simulink model "NM100A_MotVelCtrl"  (R2013b)
settings: Solver=FixedStepDiscrete  SolverMode=SingleTasking  StartTime=0.0  StopTime=1  FixedStep=0.002  RelTol=1e-3
values from neighbouring files (symbols this model uses):
  ARCHGLBPRM_2MILLISEC_SEC_F32 = DataDict.Constant    [NM100A_MotVelCtrl_DataDict.m]
  DERIVTVLPFILTICONLOWRLIM_SEC_F32 = DataDict.Constant    [NM100A_MotVelCtrl_DataDict.m]
  FALSE_CNT_LGC = DataDict.Constant    [NM100A_MotVelCtrl_DataDict.m]
  MOTVELTHDRAMPDWNCMPL_MOTRADPERSEC_F32 = DataDict.Constant    [NM100A_MotVelCtrl_DataDict.m]
  ONEMILLISEC_SEC_F32 = DataDict.Constant    [NM100A_MotVelCtrl_DataDict.m]
  TITHDRAMPDWNCMPL_CNT_U16 = DataDict.Constant    [NM100A_MotVelCtrl_DataDict.m]
  TRUE_CNT_LGC = DataDict.Constant    [NM100A_MotVelCtrl_DataDict.m]
  ZEROMOTVELTAR_MOTRADPERSEC_F32 = DataDict.Constant    [NM100A_MotVelCtrl_DataDict.m]
  ZEROTQCMD_MOTNWTMTR_F32 = DataDict.Constant    [NM100A_MotVelCtrl_DataDict.m]
libraries: NxtrLim x13, simulink x1, NxtrAbslt x1, NxtrMax x1
(part 2 of 4)

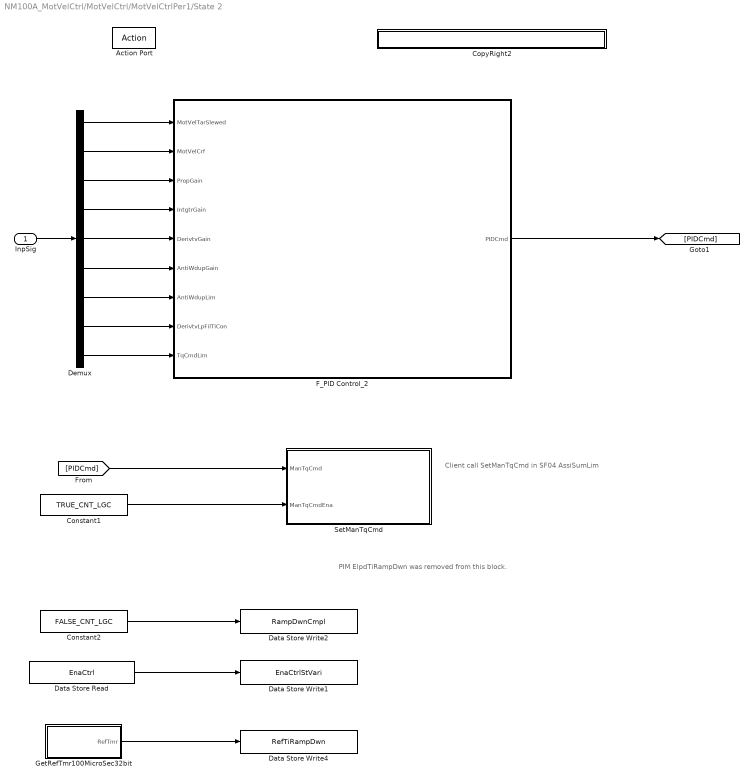
== system NM100A_MotVelCtrl/MotVelCtrl/MotVelCtrlPer1/State 2 ==
  note: PIM ElpdTiRampDwn was removed from this block.
  note: Client call SetManTqCmd in SF04 AssiSumLim
  "InpSig " : Inport
  Action Port : ActionPort  ActionType=elseif
  Constant1 : Constant  RequirementInfo="{'linktype_rmi_doors' '00010020 (/E-STEER Core/SubSystem Specifications/Manufacturing Service/NM100A_Motor Velocity Control Function Requirement)' '#NM100A_49' 'true' 'REQ:  NM100A_49' '' } %GIDa_befda8d9_aa94_48ad_b962_3d809fb1409c"  Value=TRUE_CNT_LGC
  Constant2 : Constant  RequirementInfo="{'linktype_rmi_doors' '00010020 (/E-STEER Core/SubSystem Specifications/Manufacturing Service/NM100A_Motor Velocity Control Function Requirement)' '#NM100A_49' 'true' 'REQ:  NM100A_49' '' } %GIDa_4dd34f10_b749_44c9_b696_3da1388302c2"  Value=FALSE_CNT_LGC
  CopyRight2 : Subsystem  Description=|  mask(Copyright Information){none=on}
      | Copyright info block.                                               
      |                                                                     
      | Place copyright information at the top of every subsystem in design.
      mask prompts: none "No parameters"
      mask help: Place copyright information at the top of every subsystem in design.
      mask Display:
      | NxtrConf = 'Nexteer Confidential';
      | 
      | sys = bdroot; %handle for the current model ("system")
      | first = get_param(sys,'Created');
      | if(isempty(first))
      |     first = datestr(now,'yyyy');
      | else
      |     first = first(end-3:end);  %year is last four digits
      | end
      | 
      | last = get_param(sys,'LastModifiedDate');
      | if isempty(last)
      |     last = datestr(now,'yyyy');
      | else
      |     last = last(end-3:end);
      | end
      | 
      | if strcmp(first,last)
      |     fprintf('%s -- Copyright %s Nexteer',NxtrConf,first)
      | else
      |     fprintf('%s -- %s%s- %s Nexteer',NxtrConf,char(169),first,last)
      | end
  Data Store Read : DataStoreRead  RequirementInfo={} %GIDa_be0bc7da_d338_4404_a31b_81b9c0ca05c9  DataStoreName=EnaCtrl
  Data Store Write1 : DataStoreWrite  RequirementInfo={} %GIDa_9c211729_4960_4e3d_a14f_2673763a524a  DataStoreName=EnaCtrlStVari
  Data Store Write2 : DataStoreWrite  RequirementInfo="{'linktype_rmi_doors' '00010020 (/E-STEER Core/SubSystem Specifications/Manufacturing Service/NM100A_Motor Velocity Control Function Requirement)' '#NM100A_49' 'true' 'REQ:  NM100A_49' '' ; 'linktype_rmi_doors' '00010020 (/E-STEER Core/SubSystem Specifications/Manufacturing Service/NM100A_Motor Velocity Control Function Requirement)' '#NM100A_49' 'true' 'REQ:  NM100A_49' '' } %GIDa_77af4ed3_6787_4830_bfc0_e32d42128aa7"  DataStoreName=RampDwnCmpl
  Data Store Write4 : DataStoreWrite  RequirementInfo="{'linktype_rmi_doors' '00010020 (/E-STEER Core/SubSystem Specifications/Manufacturing Service/NM100A_Motor Velocity Control Function Requirement)' '#NM100A_49' 'true' 'REQ:  NM100A_49' '' } %GIDa_d0b5b3f8_5505_4299_b70c_b09a5e077bdf"  DataStoreName=RefTiRampDwn
  Demux : Demux  Outputs=9
  F_PID Control_2 : Subsystem
  GetRefTmr100MicroSec32bit : Subsystem  RequirementInfo="{'linktype_rmi_doors' '00010020 (/E-STEER Core/SubSystem Specifications/Manufacturing Service/NM100A_Motor Velocity Control Function Requirement)' '#NM100A_49' 'true' 'REQ:  NM100A_49' '' } %GIDa_d3dda55e_dd8c_4cb5_ad41_cdb42cb83704"
  SetManTqCmd : Subsystem  RequirementInfo={} %GIDa_d5276b83_f182_4895_b3b8_b6924f7a4ac8
  wires:
  Data Store Read/1 -> Data Store Write1/1
  Constant1/1 -> SetManTqCmd/2(ManTqCmdEna)
  [PIDCmd] -> SetManTqCmd/1(ManTqCmd)
  Constant2/1 -> Data Store Write2/1
  GetRefTmr100MicroSec32bit/1(RefTmr) -> Data Store Write4/1
  F_PID Control_2/1("PIDCmd ") -> [PIDCmd]
  "InpSig "/1 -> Demux/1
  Demux/9 -> F_PID Control_2/9(TqCmdLim)
  Demux/8 -> F_PID Control_2/8(DerivtvLpFilTiCon)
  Demux/1 -> F_PID Control_2/1(MotVelTarSlewed)
  Demux/2 -> F_PID Control_2/2(MotVelCrf)
  Demux/3 -> F_PID Control_2/3(PropGain)
  Demux/4 -> F_PID Control_2/4(IntgtrGain)
  Demux/5 -> F_PID Control_2/5(DerivtvGain)
  Demux/6 -> F_PID Control_2/6(AntiWdupGain)
  Demux/7 -> F_PID Control_2/7(AntiWdupLim)

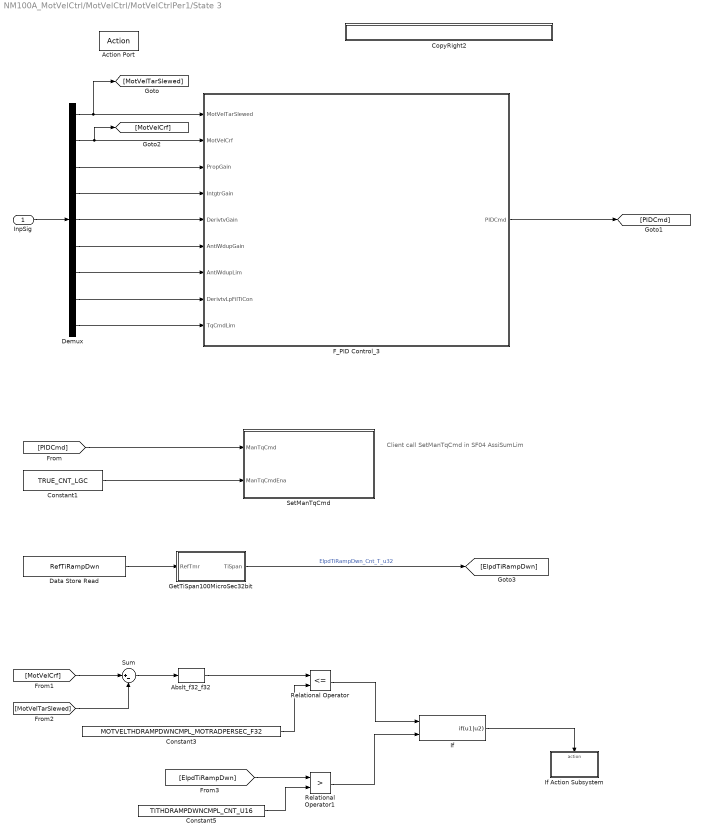
== system NM100A_MotVelCtrl/MotVelCtrl/MotVelCtrlPer1/State 3 ==
  note: Client call SetManTqCmd in SF04 AssiSumLim
  "InpSig " : Inport
  Action Port : ActionPort  ActionType=elseif
  Abslt_f32_f32 : NxtrAbslt/Abslt_f32_f32  RequirementInfo="{'linktype_rmi_doors' '00010020 (/E-STEER Core/SubSystem Specifications/Manufacturing Service/NM100A_Motor Velocity Control Function Requirement)' '#NM100A_102' 'true' 'REQ:  NM100A_102' '' } %GIDa_71536a81_3999_4725_b831_59cc761146c6"  SFunctionSpec=single y1 = Abslt_f32_f32(single u1)
      settings: AttributesFormatString=%<Name>
  Constant1 : Constant  RequirementInfo="{'linktype_rmi_doors' '00010020 (/E-STEER Core/SubSystem Specifications/Manufacturing Service/NM100A_Motor Velocity Control Function Requirement)' '#NM100A_51' 'true' 'REQ:  NM100A_51' '' } %GIDa_145580c1_2ef8_4b58_be2f_cd9335f096b6"  Value=TRUE_CNT_LGC
  Constant3 : Constant  RequirementInfo="{'linktype_rmi_doors' '00010020 (/E-STEER Core/SubSystem Specifications/Manufacturing Service/NM100A_Motor Velocity Control Function Requirement)' '#NM100A_102' 'true' 'REQ:  NM100A_102' '' } %GIDa_e1d28c76_b859_4531_ad36_30c270ff2bb5"  Value=MOTVELTHDRAMPDWNCMPL_MOTRADPERSEC_F32
  Constant5 : Constant  RequirementInfo="{'linktype_rmi_doors' '00010020 (/E-STEER Core/SubSystem Specifications/Manufacturing Service/NM100A_Motor Velocity Control Function Requirement)' '#NM100A_102' 'true' 'REQ:  NM100A_102' '' } %GIDa_b4be8dec_013e_43ed_818c_6b151e6f5195"  Value=TITHDRAMPDWNCMPL_CNT_U16
  CopyRight2 : Subsystem  Description=|  mask(Copyright Information){none=on}
      | Copyright info block.                                               
      |                                                                     
      | Place copyright information at the top of every subsystem in design.
      mask prompts: none "No parameters"
      mask help: Place copyright information at the top of every subsystem in design.
      mask Display:
      | NxtrConf = 'Nexteer Confidential';
      | 
      | sys = bdroot; %handle for the current model ("system")
      | first = get_param(sys,'Created');
      | if(isempty(first))
      |     first = datestr(now,'yyyy');
      | else
      |     first = first(end-3:end);  %year is last four digits
      | end
      | 
      | last = get_param(sys,'LastModifiedDate');
      | if isempty(last)
      |     last = datestr(now,'yyyy');
      | else
      |     last = last(end-3:end);
      | end
      | 
      | if strcmp(first,last)
      |     fprintf('%s -- Copyright %s Nexteer',NxtrConf,first)
      | else
      |     fprintf('%s -- %s%s- %s Nexteer',NxtrConf,char(169),first,last)
      | end
  Data Store Read : DataStoreRead  RequirementInfo="{'linktype_rmi_doors' '00010020 (/E-STEER Core/SubSystem Specifications/Manufacturing Service/NM100A_Motor Velocity Control Function Requirement)' '#NM100A_51' 'true' 'REQ:  NM100A_51' '' } %GIDa_01a06484_7057_4d5d_9dfb_f9d8c90e0876"  DataStoreName=RefTiRampDwn
  Demux : Demux  Outputs=9
  F_PID Control_3 : Subsystem
  GetTiSpan100MicroSec32bit : Subsystem  RequirementInfo="{'linktype_rmi_doors' '00010020 (/E-STEER Core/SubSystem Specifications/Manufacturing Service/NM100A_Motor Velocity Control Function Requirement)' '#NM100A_51' 'true' 'REQ:  NM100A_51' '' } %GIDa_c327af38_75a4_49ae_9dcc_6e10e32790a8"
  If : If  RequirementInfo="{'linktype_rmi_doors' '00010020 (/E-STEER Core/SubSystem Specifications/Manufacturing Service/NM100A_Motor Velocity Control Function Requirement)' '#NM100A_102' 'true' 'REQ:  NM100A_102' '' } %GIDa_380769d0_dc6b_456e_a037_bb1d2f196c72"  NumInputs=2  IfExpression=u1|u2  ShowElse=off
  If Action Subsystem : Subsystem  RequirementInfo="{'linktype_rmi_doors' '00010020 (/E-STEER Core/SubSystem Specifications/Manufacturing Service/NM100A_Motor Velocity Control Function Requirement)' '#NM100A_102' 'true' 'REQ:  NM100A_102' '' } %GIDa_fba956b4_c918_457d_ab20_4a25f3a425a7"  TreatAsAtomicUnit=on
  Relational Operator : RelationalOperator  RequirementInfo="{'linktype_rmi_doors' '00010020 (/E-STEER Core/SubSystem Specifications/Manufacturing Service/NM100A_Motor Velocity Control Function Requirement)' '#NM100A_102' 'true' 'REQ:  NM100A_102' '' } %GIDa_1c0824c1_3317_422e_9fa2_aea2872f56e4"  Operator=<=  OutDataTypeStr=boolean
  Relational Operator1 : RelationalOperator  RequirementInfo="{'linktype_rmi_doors' '00010020 (/E-STEER Core/SubSystem Specifications/Manufacturing Service/NM100A_Motor Velocity Control Function Requirement)' '#NM100A_102' 'true' 'REQ:  NM100A_102' '' } %GIDa_87284f63_b176_4ff1_b10d_fd7dc0737078"  Operator=>  OutDataTypeStr=boolean
  SetManTqCmd : Subsystem  RequirementInfo={} %GIDa_e23fb978_d226_45a3_bc03_4908240c5a9f
  Sum : Sum  RequirementInfo="{'linktype_rmi_doors' '00010020 (/E-STEER Core/SubSystem Specifications/Manufacturing Service/NM100A_Motor Velocity Control Function Requirement)' '#NM100A_102' 'true' 'REQ:  NM100A_102' '' } %GIDa_50c60e5b_59b9_4476_b7b5_e8ccd2770148"  Inputs=|+-
  wires:
  GetTiSpan100MicroSec32bit/1(TiSpan) -> [ElpdTiRampDwn]  "ElpdTiRampDwn_Cnt_T_u32"
  Data Store Read/1 -> GetTiSpan100MicroSec32bit/1(RefTmr)
  [MotVelCrf] -> Sum/1
  [MotVelTarSlewed] -> Sum/2
  Sum/1 -> Abslt_f32_f32/1
  Abslt_f32_f32/1 -> Relational Operator/1
  Constant3/1 -> Relational Operator/2
  [ElpdTiRampDwn] -> Relational Operator1/1
  Constant5/1 -> Relational Operator1/2
  Relational Operator/1 -> If/1
  Relational Operator1/1 -> If/2
  If/1 -> If Action Subsystem/Action
  [PIDCmd] -> SetManTqCmd/1(ManTqCmd)
  Constant1/1 -> SetManTqCmd/2(ManTqCmdEna)
  F_PID Control_3/1("PIDCmd ") -> [PIDCmd]
  "InpSig "/1 -> Demux/1
  Demux/9 -> F_PID Control_3/9(TqCmdLim)
  Demux/8 -> F_PID Control_3/8(DerivtvLpFilTiCon)
  Demux/1 -> [MotVelTarSlewed], F_PID Control_3/1(MotVelTarSlewed)
  Demux/2 -> [MotVelCrf], F_PID Control_3/2(MotVelCrf)
  Demux/3 -> F_PID Control_3/3(PropGain)
  Demux/4 -> F_PID Control_3/4(IntgtrGain)
  Demux/5 -> F_PID Control_3/5(DerivtvGain)
  Demux/6 -> F_PID Control_3/6(AntiWdupGain)
  Demux/7 -> F_PID Control_3/7(AntiWdupLim)

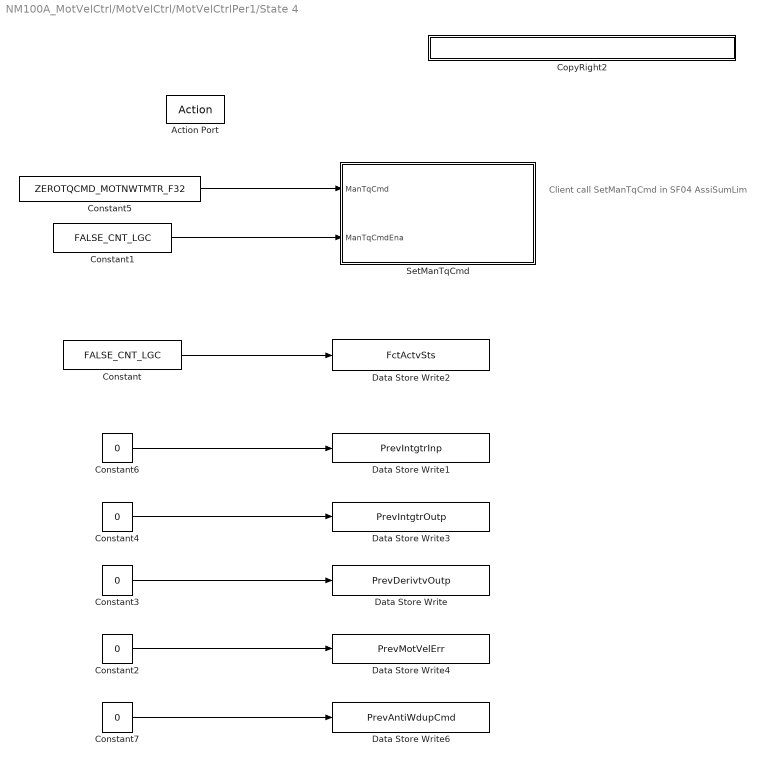
== system NM100A_MotVelCtrl/MotVelCtrl/MotVelCtrlPer1/State 4 ==
  note: Client call SetManTqCmd in SF04 AssiSumLim
  Action Port : ActionPort  ActionType=elseif
  Constant : Constant  RequirementInfo="{'linktype_rmi_doors' '00010020 (/E-STEER Core/SubSystem Specifications/Manufacturing Service/NM100A_Motor Velocity Control Function Requirement)' '#NM100A_103' 'true' 'REQ:  NM100A_103' '' } %GIDa_e0af5cdd_08fc_4257_96fd_548f729c1ff8"  Value=FALSE_CNT_LGC
  Constant1 : Constant  RequirementInfo="{'linktype_rmi_doors' '00010020 (/E-STEER Core/SubSystem Specifications/Manufacturing Service/NM100A_Motor Velocity Control Function Requirement)' '#NM100A_103' 'true' 'REQ:  NM100A_103' '' } %GIDa_4a98490f_aa1d_4f3d_87f2_701335d2a890"  Value=FALSE_CNT_LGC
  Constant2 : Constant  RequirementInfo="{'linktype_rmi_doors' '00010020 (/E-STEER Core/SubSystem Specifications/Manufacturing Service/NM100A_Motor Velocity Control Function Requirement)' '#NM100A_132' 'true' 'REQ:  NM100A_132' '' } %GIDa_c08df92f_5a02_4e06_8009_e26f95953966"  Value=0  OutDataTypeStr=single
  Constant3 : Constant  RequirementInfo="{'linktype_rmi_doors' '00010020 (/E-STEER Core/SubSystem Specifications/Manufacturing Service/NM100A_Motor Velocity Control Function Requirement)' '#NM100A_132' 'true' 'REQ:  NM100A_132' '' } %GIDa_74271fdc_8687_4593_ab71_e98823fce526"  Value=0  OutDataTypeStr=single
  Constant4 : Constant  RequirementInfo="{'linktype_rmi_doors' '00010020 (/E-STEER Core/SubSystem Specifications/Manufacturing Service/NM100A_Motor Velocity Control Function Requirement)' '#NM100A_132' 'true' 'REQ:  NM100A_132' '' } %GIDa_5f8c01d9_33ff_4742_87ff_920fa99edd06"  Value=0  OutDataTypeStr=single
  Constant5 : Constant  RequirementInfo="{'linktype_rmi_doors' '00010020 (/E-STEER Core/SubSystem Specifications/Manufacturing Service/NM100A_Motor Velocity Control Function Requirement)' '#NM100A_103' 'true' 'REQ:  NM100A_103' '' } %GIDa_14e8f590_79a8_40b3_b671_09126d55396b"  Value=ZEROTQCMD_MOTNWTMTR_F32
  Constant6 : Constant  RequirementInfo="{'linktype_rmi_doors' '00010020 (/E-STEER Core/SubSystem Specifications/Manufacturing Service/NM100A_Motor Velocity Control Function Requirement)' '#NM100A_132' 'true' 'REQ:  NM100A_132' '' } %GIDa_6c204c9d_6218_436f_9ecb_c10029247157"  Value=0  OutDataTypeStr=single
  Constant7 : Constant  RequirementInfo="{'linktype_rmi_doors' '00010020 (/E-STEER Core/SubSystem Specifications/Manufacturing Service/NM100A_Motor Velocity Control Function Requirement)' '#NM100A_132' 'true' 'REQ:  NM100A_132' '' } %GIDa_c396e5c7_5d94_4e94_a666_aede99a7520f"  Value=0  OutDataTypeStr=single
  CopyRight2 : Subsystem  Description=|  mask(Copyright Information){none=on}
      | Copyright info block.                                               
      |                                                                     
      | Place copyright information at the top of every subsystem in design.
      mask prompts: none "No parameters"
      mask help: Place copyright information at the top of every subsystem in design.
      mask Display:
      | NxtrConf = 'Nexteer Confidential';
      | 
      | sys = bdroot; %handle for the current model ("system")
      | first = get_param(sys,'Created');
      | if(isempty(first))
      |     first = datestr(now,'yyyy');
      | else
      |     first = first(end-3:end);  %year is last four digits
      | end
      | 
      | last = get_param(sys,'LastModifiedDate');
      | if isempty(last)
      |     last = datestr(now,'yyyy');
      | else
      |     last = last(end-3:end);
      | end
      | 
      | if strcmp(first,last)
      |     fprintf('%s -- Copyright %s Nexteer',NxtrConf,first)
      | else
      |     fprintf('%s -- %s%s- %s Nexteer',NxtrConf,char(169),first,last)
      | end
  Data Store Write : DataStoreWrite  RequirementInfo="{'linktype_rmi_doors' '00010020 (/E-STEER Core/SubSystem Specifications/Manufacturing Service/NM100A_Motor Velocity Control Function Requirement)' '#NM100A_132' 'true' 'REQ:  NM100A_132' '' } %GIDa_d60505be_a89c_40ef_ad23_4df5d7d8441f"  DataStoreName=PrevDerivtvOutp
  Data Store Write1 : DataStoreWrite  RequirementInfo="{'linktype_rmi_doors' '00010020 (/E-STEER Core/SubSystem Specifications/Manufacturing Service/NM100A_Motor Velocity Control Function Requirement)' '#NM100A_132' 'true' 'REQ:  NM100A_132' '' } %GIDa_90c6de6d_b636_45fd_be9c_0bef990974b9"  DataStoreName=PrevIntgtrInp
  Data Store Write2 : DataStoreWrite  RequirementInfo="{'linktype_rmi_doors' '00010020 (/E-STEER Core/SubSystem Specifications/Manufacturing Service/NM100A_Motor Velocity Control Function Requirement)' '#NM100A_103' 'true' 'REQ:  NM100A_103' '' } %GIDa_ce885f20_d047_4a81_96f7_7d088f6c7471"  DataStoreName=FctActvSts
  Data Store Write3 : DataStoreWrite  RequirementInfo="{'linktype_rmi_doors' '00010020 (/E-STEER Core/SubSystem Specifications/Manufacturing Service/NM100A_Motor Velocity Control Function Requirement)' '#NM100A_132' 'true' 'REQ:  NM100A_132' '' } %GIDa_cc8f8250_d580_4b1e_ba1d_46df9b018bff"  DataStoreName=PrevIntgtrOutp
  Data Store Write4 : DataStoreWrite  RequirementInfo="{'linktype_rmi_doors' '00010020 (/E-STEER Core/SubSystem Specifications/Manufacturing Service/NM100A_Motor Velocity Control Function Requirement)' '#NM100A_132' 'true' 'REQ:  NM100A_132' '' } %GIDa_fa392152_1c2a_4bda_84e9_c453589a09fe"  DataStoreName=PrevMotVelErr
  Data Store Write6 : DataStoreWrite  RequirementInfo="{'linktype_rmi_doors' '00010020 (/E-STEER Core/SubSystem Specifications/Manufacturing Service/NM100A_Motor Velocity Control Function Requirement)' '#NM100A_132' 'true' 'REQ:  NM100A_132' '' } %GIDa_e967ece6_5ffc_46ce_86f4_378f565c98d6"  DataStoreName=PrevAntiWdupCmd
  SetManTqCmd : Subsystem  RequirementInfo={} %GIDa_c501183d_31f0_413c_9518_9aa274485215
  wires:
  Constant/1 -> Data Store Write2/1
  Constant5/1 -> SetManTqCmd/1(ManTqCmd)
  Constant1/1 -> SetManTqCmd/2(ManTqCmdEna)
  Constant2/1 -> Data Store Write4/1
  Constant3/1 -> Data Store Write/1
  Constant4/1 -> Data Store Write3/1
  Constant6/1 -> Data Store Write1/1
  Constant7/1 -> Data Store Write6/1

== system NM100A_MotVelCtrl/MotVelCtrl/MotVelCtrlPer1/State 5 Do Nothing ==
  note: Wait and do nothing in this state.
  Action Port : ActionPort  ActionType=else
  CopyRight2 : Subsystem  Description=|  mask(Copyright Information){none=on}
      | Copyright info block.                                               
      |                                                                     
      | Place copyright information at the top of every subsystem in design.
      mask prompts: none "No parameters"
      mask help: Place copyright information at the top of every subsystem in design.
      mask Display:
      | NxtrConf = 'Nexteer Confidential';
      | 
      | sys = bdroot; %handle for the current model ("system")
      | first = get_param(sys,'Created');
      | if(isempty(first))
      |     first = datestr(now,'yyyy');
      | else
      |     first = first(end-3:end);  %year is last four digits
      | end
      | 
      | last = get_param(sys,'LastModifiedDate');
      | if isempty(last)
      |     last = datestr(now,'yyyy');
      | else
      |     last = last(end-3:end);
      | end
      | 
      | if strcmp(first,last)
      |     fprintf('%s -- Copyright %s Nexteer',NxtrConf,first)
      | else
      |     fprintf('%s -- %s%s- %s Nexteer',NxtrConf,char(169),first,last)
      | end

== system NM100A_MotVelCtrl/MotVelCtrl/SetCtrlPrm/CopyRight2 ==

== system NM100A_MotVelCtrl/MotVelCtrl/StopCtrl/CopyRight2 ==

== system NM100A_MotVelCtrl/MotVelCtrl/StrtCtrl/CopyRight2 ==

== system NM100A_MotVelCtrl/MotVelCtrl/MotVelCtrlPer1/SlewMotVelTar/CopyRight2 ==

== system NM100A_MotVelCtrl/MotVelCtrl/MotVelCtrlPer1/State 1/CopyRight2 ==

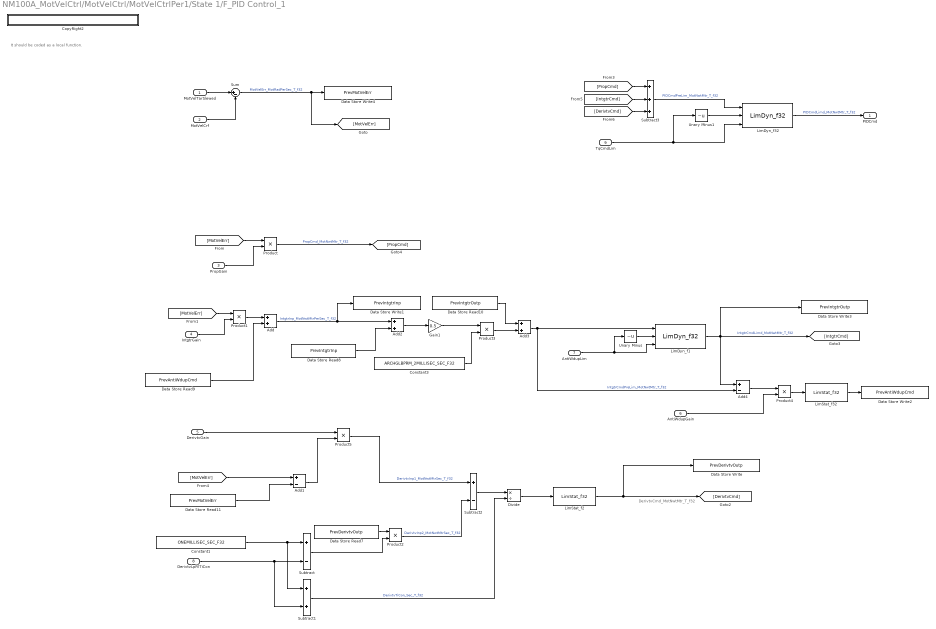
== system NM100A_MotVelCtrl/MotVelCtrl/MotVelCtrlPer1/State 1/F_PID Control_1 ==
  note: DerivtvCmd_MotNwtMtr_T_f32
  note: It should be coded as a local function.
  MotVelTarSlewed : Inport  RequirementInfo="{'linktype_rmi_doors' '00010020 (/E-STEER Core/SubSystem Specifications/Manufacturing Service/NM100A_Motor Velocity Control Function Requirement)' '#NM100A_30' 'true' 'REQ:  NM100A_30' '' } %GIDa_ba9429c3_b2a6_44fd_8328_ed63e261e922"
  MotVelCrf : Inport  RequirementInfo="{'linktype_rmi_doors' '00010020 (/E-STEER Core/SubSystem Specifications/Manufacturing Service/NM100A_Motor Velocity Control Function Requirement)' '#NM100A_30' 'true' 'REQ:  NM100A_30' '' } %GIDa_249e43ce_6396_4e5c_aa17_12a37b4ce850"  Port=2
  PropGain : Inport  RequirementInfo="{'linktype_rmi_doors' '00010020 (/E-STEER Core/SubSystem Specifications/Manufacturing Service/NM100A_Motor Velocity Control Function Requirement)' '#NM100A_112' 'true' 'REQ:  NM100A_112' '' } %GIDa_d2918d69_dd8c_483f_a043_c74a9c170ab9"  Port=3
  IntgtrGain : Inport  RequirementInfo="{'linktype_rmi_doors' '00010020 (/E-STEER Core/SubSystem Specifications/Manufacturing Service/NM100A_Motor Velocity Control Function Requirement)' '#NM100A_115' 'true' 'REQ:  NM100A_115' '' } %GIDa_bd070368_5372_458b_86f2_5ff06bf43677"  Port=4
  DerivtvGain : Inport  RequirementInfo="{'linktype_rmi_doors' '00010020 (/E-STEER Core/SubSystem Specifications/Manufacturing Service/NM100A_Motor Velocity Control Function Requirement)' '#NM100A_116' 'true' 'REQ:  NM100A_116' '' } %GIDa_947ca68e_fedf_47ef_844e_2f43d2f7ba60"  Port=5
  AntiWdupGain : Inport  RequirementInfo="{'linktype_rmi_doors' '00010020 (/E-STEER Core/SubSystem Specifications/Manufacturing Service/NM100A_Motor Velocity Control Function Requirement)' '#NM100A_118' 'true' 'REQ:  NM100A_118' '' } %GIDa_38b42111_2f7d_457c_8f7a_1eb8d27ba3f8"  Port=6
  AntiWdupLim : Inport  RequirementInfo="{'linktype_rmi_doors' '00010020 (/E-STEER Core/SubSystem Specifications/Manufacturing Service/NM100A_Motor Velocity Control Function Requirement)' '#NM100A_118' 'true' 'REQ:  NM100A_118' '' } %GIDa_29cfa6f2_eda7_4d1c_8a74_b9a9d786c745"  Port=7
  DerivtvLpFilTiCon : Inport  RequirementInfo="{'linktype_rmi_doors' '00010020 (/E-STEER Core/SubSystem Specifications/Manufacturing Service/NM100A_Motor Velocity Control Function Requirement)' '#NM100A_116' 'true' 'REQ:  NM100A_116' '' } %GIDa_5626f835_1586_4d6d_8f6e_8c5bf324693b"  Port=8
  TqCmdLim : Inport  RequirementInfo="{'linktype_rmi_doors' '00010020 (/E-STEER Core/SubSystem Specifications/Manufacturing Service/NM100A_Motor Velocity Control Function Requirement)' '#NM100A_123' 'true' 'REQ:  NM100A_123' '' } %GIDa_1e3e1849_4718_4d31_8f87_cac933a70f40"  Port=9
  Add : Sum  RequirementInfo="{'linktype_rmi_doors' '00010020 (/E-STEER Core/SubSystem Specifications/Manufacturing Service/NM100A_Motor Velocity Control Function Requirement)' '#NM100A_115' 'true' 'REQ:  NM100A_115' '' } %GIDa_25a704dd_c9d1_4845_b956_997790c43ace"
  Add1 : Sum  RequirementInfo="{'linktype_rmi_doors' '00010020 (/E-STEER Core/SubSystem Specifications/Manufacturing Service/NM100A_Motor Velocity Control Function Requirement)' '#NM100A_116' 'true' 'REQ:  NM100A_116' '' } %GIDa_012f7c69_ba98_4d6b_b5f0_33cfecf4ee6d"  Inputs=+-
  Add2 : Sum  RequirementInfo="{'linktype_rmi_doors' '00010020 (/E-STEER Core/SubSystem Specifications/Manufacturing Service/NM100A_Motor Velocity Control Function Requirement)' '#NM100A_115' 'true' 'REQ:  NM100A_115' '' } %GIDa_529e6f67_8be2_4dad_9470_b5eba2f52912"
  Add3 : Sum  RequirementInfo="{'linktype_rmi_doors' '00010020 (/E-STEER Core/SubSystem Specifications/Manufacturing Service/NM100A_Motor Velocity Control Function Requirement)' '#NM100A_115' 'true' 'REQ:  NM100A_115' '' } %GIDa_50298e16_fdb3_4c99_8cdc_cd68ad835e0b"
  Add4 : Sum  RequirementInfo={'linktype_rmi_doors' '00010020 (/E-STEER Core/SubSystem Specifications/Manufacturing Service/NM100A_Motor Velocity Control Function Requirement)' '#NM100A_118' 'true' 'REQ:NM100A_118' '' } %GIDa_b87562fd_2e83_4d37_9c91_b002b33c54af  Inputs=+-
  Constant1 : Constant  RequirementInfo="{'linktype_rmi_doors' '00010020 (/E-STEER Core/SubSystem Specifications/Manufacturing Service/NM100A_Motor Velocity Control Function Requirement)' '#NM100A_116' 'true' 'REQ:  NM100A_116' '' } %GIDa_70122f75_8c90_4f57_9e0f_909ebc7f7a2c"  Value=ONEMILLISEC_SEC_F32
  Constant3 : Constant  RequirementInfo="{'linktype_rmi_doors' '00010020 (/E-STEER Core/SubSystem Specifications/Manufacturing Service/NM100A_Motor Velocity Control Function Requirement)' '#NM100A_115' 'true' 'REQ:  NM100A_115' '' } %GIDa_9527d714_8fcf_4559_8899_418ffd3a7660"  Value=ARCHGLBPRM_2MILLISEC_SEC_F32
  CopyRight2 : Subsystem  Description=|  mask(Copyright Information){none=on}
      | Copyright info block.                                               
      |                                                                     
      | Place copyright information at the top of every subsystem in design.
      mask prompts: none "No parameters"
      mask help: Place copyright information at the top of every subsystem in design.
      mask Display:
      | NxtrConf = 'Nexteer Confidential';
      | 
      | sys = bdroot; %handle for the current model ("system")
      | first = get_param(sys,'Created');
      | if(isempty(first))
      |     first = datestr(now,'yyyy');
      | else
      |     first = first(end-3:end);  %year is last four digits
      | end
      | 
      | last = get_param(sys,'LastModifiedDate');
      | if isempty(last)
      |     last = datestr(now,'yyyy');
      | else
      |     last = last(end-3:end);
      | end
      | 
      | if strcmp(first,last)
      |     fprintf('%s -- Copyright %s Nexteer',NxtrConf,first)
      | else
      |     fprintf('%s -- %s%s- %s Nexteer',NxtrConf,char(169),first,last)
      | end
  Data Store Read10 : DataStoreRead  RequirementInfo="{'linktype_rmi_doors' '00010020 (/E-STEER Core/SubSystem Specifications/Manufacturing Service/NM100A_Motor Velocity Control Function Requirement)' '#NM100A_115' 'true' 'REQ:  NM100A_115' '' } %GIDa_687aece3_9f80_466d_9de9_e3cb1ea81850"  Priority=1  DataStoreName=PrevIntgtrOutp
  Data Store Read11 : DataStoreRead  RequirementInfo="{'linktype_rmi_doors' '00010020 (/E-STEER Core/SubSystem Specifications/Manufacturing Service/NM100A_Motor Velocity Control Function Requirement)' '#NM100A_116' 'true' 'REQ:  NM100A_116' '' } %GIDa_4290bcdf_0a17_42a8_9871_b33e1ea3d554"  Priority=1  DataStoreName=PrevMotVelErr
  Data Store Read7 : DataStoreRead  RequirementInfo="{'linktype_rmi_doors' '00010020 (/E-STEER Core/SubSystem Specifications/Manufacturing Service/NM100A_Motor Velocity Control Function Requirement)' '#NM100A_116' 'true' 'REQ:  NM100A_116' '' } %GIDa_d5aac981_534e_4fe9_8c13_af2e2de1b167"  Priority=1  DataStoreName=PrevDerivtvOutp
  Data Store Read8 : DataStoreRead  RequirementInfo="{'linktype_rmi_doors' '00010020 (/E-STEER Core/SubSystem Specifications/Manufacturing Service/NM100A_Motor Velocity Control Function Requirement)' '#NM100A_115' 'true' 'REQ:  NM100A_115' '' } %GIDa_a386e5fa_5ba8_459d_b678_d402aa374cd6"  Priority=1  DataStoreName=PrevIntgtrInp
  Data Store Read9 : DataStoreRead  RequirementInfo="{'linktype_rmi_doors' '00010020 (/E-STEER Core/SubSystem Specifications/Manufacturing Service/NM100A_Motor Velocity Control Function Requirement)' '#NM100A_9' 'true' 'REQ:  NM100A_9' '' } %GIDa_431f2dba_601e_4c5e_bc15_28ba0ea75032"  Priority=1  DataStoreName=PrevAntiWdupCmd
  Data Store Write : DataStoreWrite  RequirementInfo="{'linktype_rmi_doors' '00010020 (/E-STEER Core/SubSystem Specifications/Manufacturing Service/NM100A_Motor Velocity Control Function Requirement)' '#NM100A_116' 'true' 'REQ:  NM100A_116' '' } %GIDa_903f4395_30b7_45a4_8e25_78666363afb3"  Priority=2  DataStoreName=PrevDerivtvOutp
  Data Store Write1 : DataStoreWrite  RequirementInfo="{'linktype_rmi_doors' '00010020 (/E-STEER Core/SubSystem Specifications/Manufacturing Service/NM100A_Motor Velocity Control Function Requirement)' '#NM100A_115' 'true' 'REQ:  NM100A_115' '' } %GIDa_f926c7c7_927c_4d29_b873_66dd26dedfa7"  Priority=2  DataStoreName=PrevIntgtrInp
  Data Store Write2 : DataStoreWrite  RequirementInfo="{'linktype_rmi_doors' '00010020 (/E-STEER Core/SubSystem Specifications/Manufacturing Service/NM100A_Motor Velocity Control Function Requirement)' '#NM100A_118' 'true' 'REQ:  NM100A_118' '' } %GIDa_26a96735_57eb_474e_858a_037ac73c1f93"  Priority=2  DataStoreName=PrevAntiWdupCmd
  Data Store Write3 : DataStoreWrite  RequirementInfo="{'linktype_rmi_doors' '00010020 (/E-STEER Core/SubSystem Specifications/Manufacturing Service/NM100A_Motor Velocity Control Function Requirement)' '#NM100A_115' 'true' 'REQ:  NM100A_115' '' } %GIDa_c8af5739_c4f1_481c_ad29_186d536bef69"  Priority=2  DataStoreName=PrevIntgtrOutp
  Data Store Write4 : DataStoreWrite  RequirementInfo="{'linktype_rmi_doors' '00010020 (/E-STEER Core/SubSystem Specifications/Manufacturing Service/NM100A_Motor Velocity Control Function Requirement)' '#NM100A_30' 'true' 'REQ:  NM100A_30' '' } %GIDa_2b6a2ba6_564a_4289_8c64_4b6d19a43dc4"  Priority=2  DataStoreName=PrevMotVelErr
  Divide : Product  RequirementInfo="{'linktype_rmi_doors' '00010020 (/E-STEER Core/SubSystem Specifications/Manufacturing Service/NM100A_Motor Velocity Control Function Requirement)' '#NM100A_116' 'true' 'REQ:  NM100A_116' '' } %GIDa_20cf7746_3cae_4202_9f0a_8f463bab2326"  Inputs=*/
  Gain1 : Gain  RequirementInfo="{'linktype_rmi_doors' '00010020 (/E-STEER Core/SubSystem Specifications/Manufacturing Service/NM100A_Motor Velocity Control Function Requirement)' '#NM100A_115' 'true' 'REQ:  NM100A_115' '' } %GIDa_2ca42ec1_bc27_470e_badd_555b4de840b5"  Gain=0.5  ParamDataTypeStr=single  OutDataTypeStr=single
  LimDyn_f1 : NxtrLim/LimDyn_f32  RequirementInfo="{'linktype_rmi_doors' '00010020 (/E-STEER Core/SubSystem Specifications/Manufacturing Service/NM100A_Motor Velocity Control Function Requirement)' '#NM100A_115' 'true' 'REQ:  NM100A_115' '' ; 'linktype_rmi_doors' '00010020 (/E-STEER Core/SubSystem Specifications/Manufacturing Service/NM100A_Motor Velocity Control Function Requirement)' '#NM100A_118' 'true' 'REQ:  NM100A_118' '' } %GIDa_cb727b3a_0fa7_46b8_9e48_e249cad81d32"
  LimDyn_f32 : NxtrLim/LimDyn_f32  RequirementInfo="{'linktype_rmi_doors' '00010020 (/E-STEER Core/SubSystem Specifications/Manufacturing Service/NM100A_Motor Velocity Control Function Requirement)' '#NM100A_123' 'true' 'REQ:  NM100A_123' '' } %GIDa_d4111f85_207a_4526_9ec5_9a4a393dc94e"
  LimStat_f2 : NxtrLim/LimStat_f32  RequirementInfo={'linktype_rmi_doors' '00010020 (/E-STEER Core/SubSystem Specifications/Manufacturing Service/NM100A_Motor Velocity Control Function Requirement)' '#NM100A_116' 'true' 'REQ:NM100A_116' '' } %GIDa_3b6b9b3f_0ade_4cbd_9da4_70d0e1196e4c  LoLim=DERIVTVCMDLOWRLIM_MOTNWTMTR_F32  HiLim=DERIVTVCMDUPPRLIM_MOTNWTMTR_F32
      settings: AttributesFormatString=|
      | Low Limit: %<LoLim>
      | High Limit:%<HiLim>
  LimStat_f32 : NxtrLim/LimStat_f32  RequirementInfo={'linktype_rmi_doors' '00010020 (/E-STEER Core/SubSystem Specifications/Manufacturing Service/NM100A_Motor Velocity Control Function Requirement)' '#NM100A_118' 'true' 'REQ:NM100A_118' '' } %GIDa_10ac2318_83d0_488c_bf42_b067ebb89913  LoLim=ANTIWDUPCMDLOWRLIM_MOTNWTMTR_F32  HiLim=ANTIWDUPCMDUPPRLIM_MOTNWTMTR_F32
      settings: AttributesFormatString=|
      | Low Limit: %<LoLim>
      | High Limit:%<HiLim>
  Product : Product  RequirementInfo="{'linktype_rmi_doors' '00010020 (/E-STEER Core/SubSystem Specifications/Manufacturing Service/NM100A_Motor Velocity Control Function Requirement)' '#NM100A_112' 'true' 'REQ:  NM100A_112' '' } %GIDa_30a037a1_fa70_485e_8905_69686eb1391e"
  Product1 : Product  RequirementInfo="{'linktype_rmi_doors' '00010020 (/E-STEER Core/SubSystem Specifications/Manufacturing Service/NM100A_Motor Velocity Control Function Requirement)' '#NM100A_115' 'true' 'REQ:  NM100A_115' '' } %GIDa_660da590_1a2d_482e_82a6_627b75253ff1"
  Product2 : Product  RequirementInfo="{'linktype_rmi_doors' '00010020 (/E-STEER Core/SubSystem Specifications/Manufacturing Service/NM100A_Motor Velocity Control Function Requirement)' '#NM100A_116' 'true' 'REQ:  NM100A_116' '' } %GIDa_c85576af_6643_47b3_80a9_562ae4eddf56"
  Product3 : Product  RequirementInfo="{'linktype_rmi_doors' '00010020 (/E-STEER Core/SubSystem Specifications/Manufacturing Service/NM100A_Motor Velocity Control Function Requirement)' '#NM100A_115' 'true' 'REQ:  NM100A_115' '' } %GIDa_3a770359_88a4_4cac_aa32_e199e6a903e3"
  Product4 : Product  RequirementInfo={'linktype_rmi_doors' '00010020 (/E-STEER Core/SubSystem Specifications/Manufacturing Service/NM100A_Motor Velocity Control Function Requirement)' '#NM100A_118' 'true' 'REQ:NM100A_118' '' } %GIDa_de214d40_dc05_40d7_b8ba_3a8fc90753c4
  Product5 : Product  RequirementInfo="{'linktype_rmi_doors' '00010020 (/E-STEER Core/SubSystem Specifications/Manufacturing Service/NM100A_Motor Velocity Control Function Requirement)' '#NM100A_116' 'true' 'REQ:  NM100A_116' '' } %GIDa_477657a9_ade9_4784_ad08_1ce606cc5767"
  Subtract : Sum  RequirementInfo="{'linktype_rmi_doors' '00010020 (/E-STEER Core/SubSystem Specifications/Manufacturing Service/NM100A_Motor Velocity Control Function Requirement)' '#NM100A_116' 'true' 'REQ:  NM100A_116' '' } %GIDa_1dceebc2_6e2c_434c_a6fa_6565ee1f9297"  Inputs=+-
  Subtract1 : Sum  RequirementInfo="{'linktype_rmi_doors' '00010020 (/E-STEER Core/SubSystem Specifications/Manufacturing Service/NM100A_Motor Velocity Control Function Requirement)' '#NM100A_116' 'true' 'REQ:  NM100A_116' '' } %GIDa_bf63683c_0b33_4028_ad12_244ce5d42498"
  Subtract2 : Sum  RequirementInfo="{'linktype_rmi_doors' '00010020 (/E-STEER Core/SubSystem Specifications/Manufacturing Service/NM100A_Motor Velocity Control Function Requirement)' '#NM100A_116' 'true' 'REQ:  NM100A_116' '' } %GIDa_1b9fc4f6_b1a7_463b_84bc_39c7cb70b97c"  Inputs=+-
  Subtract3 : Sum  RequirementInfo="{'linktype_rmi_doors' '00010020 (/E-STEER Core/SubSystem Specifications/Manufacturing Service/NM100A_Motor Velocity Control Function Requirement)' '#NM100A_122' 'true' 'REQ:  NM100A_122' '' } %GIDa_e77d6b67_59fe_4679_b125_40452a4a685f"  Inputs=+++
  Sum : Sum  RequirementInfo="{'linktype_rmi_doors' '00010020 (/E-STEER Core/SubSystem Specifications/Manufacturing Service/NM100A_Motor Velocity Control Function Requirement)' '#NM100A_30' 'true' 'REQ:  NM100A_30' '' } %GIDa_5f3d9d75_fc10_4187_bd9c_b94e1f88334f"  Inputs=|+-
  Unary Minus : UnaryMinus  RequirementInfo="{'linktype_rmi_doors' '00010020 (/E-STEER Core/SubSystem Specifications/Manufacturing Service/NM100A_Motor Velocity Control Function Requirement)' '#NM100A_115' 'true' 'REQ:  NM100A_115' '' ; 'linktype_rmi_doors' '00010020 (/E-STEER Core/SubSystem Specifications/Manufacturing Service/NM100A_Motor Velocity Control Function Requirement)' '#NM100A_118' 'true' 'REQ:  NM100A_118' '' } %GIDa_982d5e2d_a8ad_4e37_891c_e7ef499ec766"
  Unary Minus1 : UnaryMinus  RequirementInfo="{'linktype_rmi_doors' '00010020 (/E-STEER Core/SubSystem Specifications/Manufacturing Service/NM100A_Motor Velocity Control Function Requirement)' '#NM100A_123' 'true' 'REQ:  NM100A_123' '' } %GIDa_4269fde5_8259_4b08_9e18_813eb1fe1e31"
  "PIDCmd " : Outport
  wires:
  [MotVelErr] -> Product/1
  PropGain/1 -> Product/2
  [MotVelErr] -> Product1/1
  IntgtrGain/1 -> Product1/2
  Product1/1 -> Add/1
  Data Store Read9/1 -> Add/2
  Add/1 -> Data Store Write1/1, Add2/1  "IntgtrInp_MotNwtMtrPerSec_T_f32"
  Add2/1 -> Gain1/1
  Gain1/1 -> Product3/1
  Constant3/1 -> Product3/2
  Product3/1 -> Add3/2
  Add3/1 -> Add4/2, LimDyn_f1/1  "IntgtrCmdPreLim_MotNwtMtr_T_f32"
  LimDyn_f1/1 -> Data Store Write3/1, Add4/1, [IntgtrCmd]  "IntgtrCmdLimd_MotNwtMtr_T_f32"
  AntiWdupLim/1 -> Unary Minus/1, LimDyn_f1/3
  Unary Minus/1 -> LimDyn_f1/2
  [MotVelErr] -> Add1/1
  Constant1/1 -> Subtract1/1, Subtract/1
  DerivtvLpFilTiCon/1 -> Subtract1/2, Subtract/2
  Subtract/1 -> Product2/2
  Data Store Read7/1 -> Product2/1
  Product2/1 -> Subtract2/2  "DerivtvInp2_MotNwtMtrSec_T_f32"
  Subtract2/1 -> Divide/1
  Subtract1/1 -> Divide/2  "DerivtvTiCon_Sec_T_f32"
  Product/1 -> [PropCmd]  "PropCmd_MotNwtMtr_T_f32"
  [PropCmd] -> Subtract3/1
  [IntgtrCmd] -> Subtract3/2
  [DerivtvCmd] -> Subtract3/3
  Subtract3/1 -> LimDyn_f32/1  "PIDCmdPreLim_MotNwtMtr_T_f32"
  Unary Minus1/1 -> LimDyn_f32/2
  TqCmdLim/1 -> LimDyn_f32/3, Unary Minus1/1
  LimDyn_f32/1 -> "PIDCmd "/1  "PIDCmdLimd_MotNwtMtr_T_f32"
  Divide/1 -> LimStat_f2/1
  Data Store Read8/1 -> Add2/2
  Data Store Read10/1 -> Add3/1
  Data Store Read11/1 -> Add1/2
  Sum/1 -> [MotVelErr], Data Store Write4/1  "MotVelErr_MotRadPerSec_T_f32"
  Add4/1 -> Product4/1
  AntiWdupGain/1 -> Product4/2
  DerivtvGain/1 -> Product5/1
  Add1/1 -> Product5/2
  Product5/1 -> Subtract2/1  "DerivtvInp1_MotNwtMtrSec_T_f32"
  MotVelTarSlewed/1 -> Sum/1
  MotVelCrf/1 -> Sum/2
  Product4/1 -> LimStat_f32/1
  LimStat_f32/1 -> Data Store Write2/1
  LimStat_f2/1 -> Data Store Write/1, [DerivtvCmd]

== system NM100A_MotVelCtrl/MotVelCtrl/MotVelCtrlPer1/State 1/SetManTqCmd ==
  ManTqCmd : Inport  RequirementInfo="{'linktype_rmi_doors' '00010020 (/E-STEER Core/SubSystem Specifications/Manufacturing Service/NM100A_Motor Velocity Control Function Requirement)' '#NM100A_48' 'true' 'REQ:  NM100A_48' '' } %GIDa_1799be38_3be4_4fe9_939e_7c1881642f5d"
  ManTqCmdEna : Inport  RequirementInfo="{'linktype_rmi_doors' '00010020 (/E-STEER Core/SubSystem Specifications/Manufacturing Service/NM100A_Motor Velocity Control Function Requirement)' '#NM100A_48' 'true' 'REQ:  NM100A_48' '' } %GIDa_b5acf617_5b45_43cd_a941_a1beb92a46a5"  Port=2
  CopyRight2 : Subsystem  Description=|  mask(Copyright Information){none=on}
      | Copyright info block.                                               
      |                                                                     
      | Place copyright information at the top of every subsystem in design.
      mask prompts: none "No parameters"
      mask help: Place copyright information at the top of every subsystem in design.
      mask Display:
      | NxtrConf = 'Nexteer Confidential';
      | 
      | sys = bdroot; %handle for the current model ("system")
      | first = get_param(sys,'Created');
      | if(isempty(first))
      |     first = datestr(now,'yyyy');
      | else
      |     first = first(end-3:end);  %year is last four digits
      | end
      | 
      | last = get_param(sys,'LastModifiedDate');
      | if isempty(last)
      |     last = datestr(now,'yyyy');
      | else
      |     last = last(end-3:end);
      | end
      | 
      | if strcmp(first,last)
      |     fprintf('%s -- Copyright %s Nexteer',NxtrConf,first)
      | else
      |     fprintf('%s -- %s%s- %s Nexteer',NxtrConf,char(169),first,last)
      | end
  Data Store Write : DataStoreWrite  RequirementInfo="{'linktype_rmi_doors' '00010020 (/E-STEER Core/SubSystem Specifications/Manufacturing Service/NM100A_Motor Velocity Control Function Requirement)' '#NM100A_48' 'true' 'REQ:  NM100A_48' '' } %GIDa_0cb917a5_82e9_4e92_b173_736cea733007"  DataStoreName=ManTqCmd
  Data Store Write1 : DataStoreWrite  RequirementInfo="{'linktype_rmi_doors' '00010020 (/E-STEER Core/SubSystem Specifications/Manufacturing Service/NM100A_Motor Velocity Control Function Requirement)' '#NM100A_48' 'true' 'REQ:  NM100A_48' '' } %GIDa_9603700c_17db_44ef_9f25_47ef026769db"  DataStoreName=ManTqCmdEna
  wires:
  ManTqCmd/1 -> Data Store Write/1
  ManTqCmdEna/1 -> Data Store Write1/1

== system NM100A_MotVelCtrl/MotVelCtrl/MotVelCtrlPer1/State 2/CopyRight2 ==
